simulink model "RGB_uart"  (R2020b)
settings: Solver=VariableStepAuto  StartTime=0.0  StopTime=inf  RelTol=1e-3
undefined symbols (not defined in the file): serial
libraries: instrumentlib x2
settings Model: Creator=jesus  LastModifiedBy=jesus

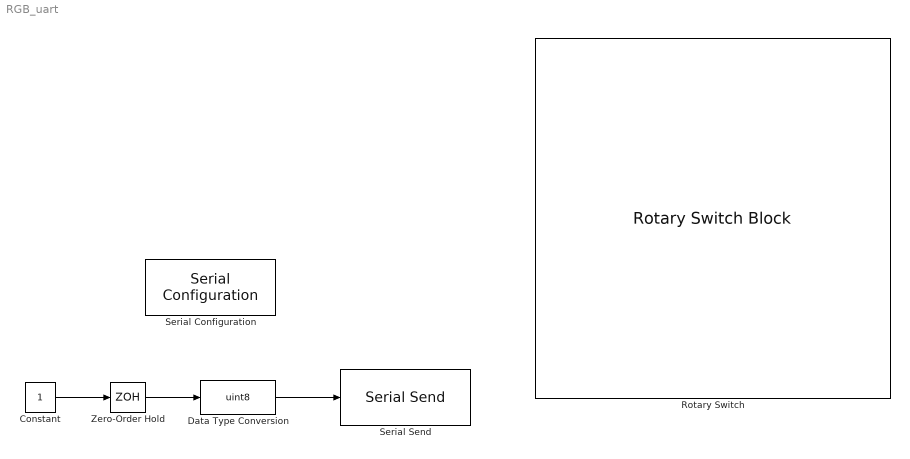
== system RGB_uart ==
  Constant : Constant
  Data Type Conversion : DataTypeConversion  OutDataTypeStr=uint8
  Rotary Switch : RotarySwitchBlock
      settings: Values={{'Off', 'Low', 'Medio', 'High', 'Rojo', 'hreen', 'Azul'}, [1 25 50 100 114 103 98]}
  Serial Configuration : instrumentlib/Serial Configuration  Priority=-200000  ComPortMenu=COM7  ComPort=COM7  ObjConstructor=serial('COM7');  BaudRate=9600  DataBits=8  Parity=none  StopBits=1  FlowControl=none  Timeout=10  ByteOrder=LittleEndian
  Serial Send : instrumentlib/Serial Send  ComPortMenu=COM7  ComPort=COM7  ObjConstructor=serial('COM7');  Terminator=<none>  EnableBlockingMode=on
  Zero-Order Hold : ZeroOrderHold  SampleTime=0.5
  wires:
  Constant/1 -> Zero-Order Hold/1
  Zero-Order Hold/1 -> Data Type Conversion/1
  Data Type Conversion/1 -> Serial Send/1
